simulink model "sistema_completo"  (R2019a)
settings: Solver=VariableStepAuto  StartTime=0.0  StopTime=120  RelTol=1e-3
InitFcn:
  | parametros
values from neighbouring files (symbols this model uses):
  a_h_max = 0.75    [parametros.m]
  a_t_max = 0.8    [parametros.m]
  b_cx = 1.0e6    (= 1000000)    [parametros.m]
  b_cy = 1.0e7    (= 10000000)    [parametros.m]
  b_h_eq = 2 * ( b_hd + i_h^2*b_hm ) / (r_hd^2)    (= 31004.4444444)    [parametros.m]
  b_hb = 1.0e8    (= 100000000)    [parametros.m]
  b_hEb = 2.2e9    (= 2200000000)    [parametros.m]
  b_t = 90.0    (= 90)    [parametros.m]
  b_t_eq = Simulink.Parameter(b_t_eq)    [parametros.m]
  b_tb = 5.0e6    (= 5000000)    [parametros.m]
  b_td_eq = ( b_td + i_t^2*b_tm ) / (r_td^2)    (= 21607.2)    [parametros.m]
  b_tw = 3.0e3    (= 3000)    [parametros.m]
  b_wu = 150    [parametros.m]
  clearance_min = 2    [parametros.m]
  g = Simulink.Parameter(9.80665)    [parametros.m]
  H_c = Simulink.Parameter(2.59)    [parametros.m]
  i_h = 22.0    (= 22)    [parametros.m]
  i_t = 30.0    (= 30)    [parametros.m]
  K_cy = 1.8e9    (= 1800000000)    [parametros.m]
  K_d_h = 2*m_h_eq*xi_hc*w_hc + m_h_eq*p3_hc - b_h_eq    (= 221460.31746)    [parametros.m]
  K_d_t = 2*m_t_eq*xi_tc*w_tc + m_t_eq*p3_tc - b_t_eq.Value    [parametros.m]
  K_i_h = m_h_eq*p3_hc*w_hc^2    (= 25598.9338431)    [parametros.m]
  K_i_t = m_t_eq*p3_tc*w_tc^2    [parametros.m]
  k_p3_th = 3    [parametros.m]
  K_p_h = m_h_eq*w_hc^2 + 2*m_h_eq*xi_hc*w_hc*p3_hc    (= 112940.617295)    [parametros.m]
  K_p_t = m_t_eq*w_tc^2 + 2*m_t_eq*xi_tc*w_tc*p3_tc    [parametros.m]
  k_th = 1    [parametros.m]
  K_tw = 4.8e5    (= 480000)    [parametros.m]
  k_w_c_th = 0.7    [parametros.m]
  k_wu = 2.36e8    (= 236000000)    [parametros.m]
  l_h0 = Y_t0 - y_h0    [parametros.m]
  L_h0 = 110    [parametros.m]
  l_h_man_thresh = 1.0    (= 1)    [parametros.m]
  l_h_tol = 1.0    (= 1)    [parametros.m]
  M_c_max = 50000    [parametros.m]
  M_c_min = 2000    [parametros.m]
  m_h_eq = 2 * ( J_hd_hEb + i_h^2*J_hm_hb ) / (r_hd^2)    (= 65137.7777778)    [parametros.m]
  M_s = 15000    [parametros.m]
  M_t = Simulink.Parameter(30000)    [parametros.m]
  m_td_eq = ( J_td + i_t^2*J_tm_tb ) / (r_td^2)    (= 30000)    [parametros.m]
  N_slots = Simulink.Parameter(floor((x_t_max_oper.Value - x_t_min_oper.Value) / W_c.Value))    [parametros.m]
  overload = false    [parametros.m]
  P_h_nom = 956150    [parametros.m]
  r_hd = 0.75    [parametros.m]
  r_td = 0.50    (= 0.5)    [parametros.m]
  random_obstacles = false    [parametros.m]
  T_hb_max = 5.0e4    (= 50000)    [parametros.m]
  T_hEb_max = 1.1e6    (= 1100000)    [parametros.m]
  T_hm_MAX = 2.0e4    (= 20000)    [parametros.m]
  T_s1 = 20/1000    (= 0.02)    [parametros.m]
  T_s2 = 1/1000    (= 0.001)    [parametros.m]
  T_tb_max = 5.0e3    (= 5000)    [parametros.m]
  T_tm_max = 4.0e3    (= 4000)    [parametros.m]
  tau_hm = 1.0    (= 1)    [parametros.m]
  tau_tm = 1.0    (= 1)    [parametros.m]
  v_h_max = 3.0    (= 3)    [parametros.m]
  v_h_nom = 1.5    [parametros.m]
  v_t_max = 4.0    (= 4)    [parametros.m]
  W_c = Simulink.Parameter(2.44)    [parametros.m]
  w_hm_rated = 2 * (i_h / r_hd) * v_h_nom    (= 88)    [parametros.m]
  x_l0 = x_t0    [parametros.m]
  x_t0 = W_c.Value / 2    [parametros.m]
  x_t_man_thresh = 1.0    (= 1)    [parametros.m]
  x_t_max_emer = x_t_max_oper.Value + 1.0    [parametros.m]
  x_t_max_oper = Simulink.Parameter(50.0)    [parametros.m]
  x_t_min_emer = x_t_min_oper.Value - 1.0    [parametros.m]
  x_t_min_oper = Simulink.Parameter(-30.0)    [parametros.m]
  x_td0 = x_t0    [parametros.m]
  xi_c_th = 0.7    [parametros.m]
  y_c0_0 = Simulink.Parameter(y_c0_ship)    [parametros.m]
  y_c0_quay = 0    [parametros.m]
  y_c0_ship = -20    [parametros.m]
  y_h_max_emer = y_h_max_oper.Value + 1.0    [parametros.m]
  y_h_max_oper = Simulink.Parameter(40.0)    [parametros.m]
  y_h_min_emer = y_h_min_oper.Value - 1.0    [parametros.m]
  y_h_min_oper = Simulink.Parameter(-20.0)    [parametros.m]
  y_l0 = y_h0    [parametros.m]
  Y_t0 = 45.0    (= 45)    [parametros.m]
undefined symbols (not defined in the file or in its folder): DiscIntNeverNeededParam, F_hw, hoist, l_h, l_h_dot, sigbuilder_block, theta_l, theta_l_dot, TLK, translation, x_t_dot
libraries: simulink x10, vrlib x1
(part 2 of 2)

== system sistema_completo/Planta física/Izaje del carro/Variables de estado derivadas ==
  note: Velocidad angular del tambor
  note: Caja reductora
      | entre motor y tambor
  note: Velocidad angular del motor
  note: Velocidad de despliegue del cable de izaje
  note: Longitud de cable de izaje desplegado
  note: Posición angular del motor
  note: Caja reductora
      | entre motor y tambor
  note: Radio del tambor
  note: Radio del tambor
  note: Normalizar ángulo en
      | rango 0 a 2*pi
  note: Posición angular del tambor
  note: Altura de carro (fija)
  note: Altura de la carga sin balanceo
  l_h_dot : Inport
  l_h : Inport  Port=2
  Constant1 : Constant  Value=2*pi
  Constant2 : Constant  Value=Y_t0
  Gain1 : Gain  Gain=-2/r_hd
  Gain2 : Gain  Gain=-2/r_hd
  Gain3 : Gain  Gain=i_h
  Gain4 : Gain  Gain=i_h
  Mod2 : Math  Operator=mod  SaturateOnIntegerOverflow=on
  Sum : Sum  Inputs=+-|
  w_hm : Outport
  w_hd : Outport  Port=2
  theta_hm : Outport  Port=3
  theta_hd : Outport  Port=4
  y_h : Outport  Port=5
  wires:
  Gain1/1 -> w_hd/1, Gain3/1  "w_hd"
  l_h_dot/1 -> Gain1/1
  Gain3/1 -> w_hm/1  "w_hm"
  Gain2/1 -> theta_hd/1, Gain4/1  "theta_hd"
  l_h/1 -> Sum/2, Gain2/1
  Gain4/1 -> Mod2/1  "theta_hm_raw"
  Constant1/1 -> Mod2/2
  Mod2/1 -> theta_hm/1
  Constant2/1 -> Sum/1
  Sum/1 -> y_h/1  "y_h"

== system sistema_completo/Planta física/Traslación del carro/Fines de carrera (fijos en viga) ==
  note: Posición horizontal del carro
  note: Fin de carrera de operación de límite normal mínimo
  note: Fin de carrera de operación de límite normal máximo
  note: Fin de carrera de emergencia de límite último mínimo
  note: Fin de carrera de operación de límite último máximo
  x_t : Inport
  Compare To Constant : simulink/Logic and Bit Operations/Compare To Constant  relop=<=  const=x_t_min_oper  OutDataTypeStr=boolean
  Compare To Constant1 : simulink/Logic and Bit Operations/Compare To Constant  relop=>=  const=x_t_max_oper  OutDataTypeStr=boolean
  Compare To Constant2 : simulink/Logic and Bit Operations/Compare To Constant  relop=<=  const=x_t_min_emer  OutDataTypeStr=boolean
  Compare To Constant3 : simulink/Logic and Bit Operations/Compare To Constant  relop=>=  const=x_t_max_emer  OutDataTypeStr=boolean
  x_t_min_oper : Outport  OutDataTypeStr=boolean  PortDimensions=1  SampleTime=0
  x_t_max_oper : Outport  Port=2  OutDataTypeStr=boolean  PortDimensions=1  SampleTime=0
  x_t_min_emer : Outport  Port=3  OutDataTypeStr=boolean  PortDimensions=1  SampleTime=0
  x_t_max_emer : Outport  Port=4  OutDataTypeStr=boolean  PortDimensions=1  SampleTime=0
  wires:
  Compare To Constant2/1 -> x_t_min_emer/1
  Compare To Constant/1 -> x_t_min_oper/1
  Compare To Constant1/1 -> x_t_max_oper/1
  x_t/1 -> Compare To Constant3/1, Compare To Constant2/1, Compare To Constant1/1, Compare To Constant/1
  Compare To Constant3/1 -> x_t_max_emer/1

== system sistema_completo/Planta física/Traslación del carro/Fuerza del cable del carro ==
  note: Posición de tambor del carro
  note: Velocidad del tambor del carro
  note: Posición del carro
  note: Velocidad del carro
  note: Fuerza del cable del carro
  x_td : Inport
  x_t : Inport  Port=2
  x_td_dot : Inport  Port=3
  x_t_dot : Inport  Port=4
  Gain : Gain  Gain=K_tw
  Gain1 : Gain  Gain=b_tw
  Sum2 : Sum  Inputs=+-
  Sum3 : Sum  Inputs=+-
  Sum4 : Sum
  F_tw : Outport
  wires:
  x_td_dot/1 -> Sum3/1
  x_td/1 -> Sum2/1
  x_t_dot/1 -> Sum3/2
  x_t/1 -> Sum2/2
  Sum4/1 -> F_tw/1
  Gain/1 -> Sum4/1
  Sum2/1 -> Gain/1
  Gain1/1 -> Sum4/2
  Sum3/1 -> Gain1/1

== system sistema_completo/Planta física/Traslación del carro/Fuerza motriz de tambor de carro equivalente ==
  note: Fuerza motriz de tambor
      | de carro equivalente
  note: Torque motor carro
  note: Freno eje rápido izaje
      | (operación)
  note: Estado de freno de
      | operación de carro
      | (eje rápido)
  note: Velocidad angular
      | del motor de carro
      | (eje rápido)
  T_tm : Inport
  BRK_t : Inport  Port=2  OutDataTypeStr=boolean
  w_tm : Inport  Port=3
  Constant4 : Constant  Value=-T_tb_max
  Constant5 : Constant  Value=T_tb_max
  Constant6 : Constant  Value=0
  Gain4 : Gain  Gain=i_t/r_td
  Gain7 : Gain  Gain=-b_tb
  MinMax2 : MinMax  Inputs=2
  MinMax3 : MinMax  Function=max  Inputs=2
  Sum1 : Sum  Inputs=++|
  Switch1 : Switch  Criteria=u2 ~= 0
  F_td_m_eq : Outport
  wires:
  MinMax3/1 -> MinMax2/2
  MinMax2/1 -> Switch1/3  "BRK_t = Off"
  Constant4/1 -> MinMax3/1
  T_tm/1 -> Sum1/1
  w_tm/1 -> Gain7/1
  Constant5/1 -> MinMax2/1
  Gain7/1 -> MinMax3/2
  BRK_t/1 -> Switch1/2
  Constant6/1 -> Switch1/1  "BRK_t = On"
  Sum1/1 -> Gain4/1
  Switch1/1 -> Sum1/2  "T_tb"
  Gain4/1 -> F_td_m_eq/1

== system sistema_completo/Planta física/Traslación del carro/Modulador de torque en accionamiento de carro ==
  note: Modelo de torque idealizado equivalente,
      | modelo simplificado de primer orden LTI en tiempo continuo
  note: Consigna de torque de motor de carro
  note: Torque de motor de carro
  T_tm* : Inport
  Gain1 : Gain  Gain=1/tau_tm
  Gain3 : Gain  Gain=-1
  Integrator2 : Integrator
  Limitador de torque máximo en tiempo discretizado : Subsystem
  Sum : Sum  Inputs=|++
  T_tm : Outport
  wires:
  Sum/1 -> Gain1/1
  Gain3/1 -> Sum/2
  Gain1/1 -> Integrator2/1  "T_tm_dot"
  Limitador de torque máximo en tiempo discretizado/1(T_tm_lim*) -> Sum/1  "T_tm_lim*"
  T_tm*/1 -> Limitador de torque máximo en tiempo discretizado/1(T_tm*)
  Integrator2/1 -> T_tm/1, Gain3/1  "T_tm"

== system sistema_completo/Planta física/Traslación del carro/Variables de estado derivadas ==
  note: Normalizar ángulo en
      | rango 0 a 2*pi
  note: Radio del tambor
  note: Caja reductora
      | entre motor y tambor
  note: Velocidad angular del motor del carro
  note: Velocidad de la carga sin balanceo
  note: Posición angular del motor del carro
  note: Caja reductora
      | entre motor y tambor
  note: Radio del tambor
  note: Posición horizontal
      | del tambor del carro
  x_td_dot : Inport
  x_td : Inport  Port=2
  Constant : Constant  Value=2*pi
  Gain1 : Gain  Gain=1/r_td
  Gain2 : Gain  Gain=1/r_td
  Gain3 : Gain  Gain=i_t
  Gain4 : Gain  Gain=i_t
  Mod1 : Math  Operator=mod  SaturateOnIntegerOverflow=on
  w_tm : Outport
  theta_tm : Outport  Port=2
  wires:
  Gain1/1 -> Gain3/1  "w_td"
  x_td_dot/1 -> Gain1/1
  Gain3/1 -> w_tm/1  "w_tm"
  x_td/1 -> Gain2/1
  Gain2/1 -> Gain4/1  "theta_td"
  Gain4/1 -> Mod1/1  "theta_tm_raw"
  Mod1/1 -> theta_tm/1
  Constant/1 -> Mod1/2

== system sistema_completo/Controladores de movimiento/Controladores de movimiento (Nivel 2)/Controlador de ángulo de balanceo/Des-linearización por retroalimentación ==
  note: Linearización por retroalimentación (feedback linearization)
      | F_t_eq = ( v - a ) / b
      | Siendo v la entrada virtual al sistema lineal a controlar
  m_l : Inport
  v : Inport  Port=2
  theta : Inport  Port=3
  theta_dot : Inport  Port=4
  x_t_dot : Inport  Port=5
  l_h : Inport  Port=6
  Add : Sum  Inputs=+-
  Divide : Product  Inputs=*/
  MATLAB Function : MATLAB Function  TreatAsAtomicUnit=on
  MATLAB Function1 : MATLAB Function  TreatAsAtomicUnit=on
  F_t_eq : Outport
  wires:
  Add/1 -> Divide/1
  v/1 -> Add/1
  Divide/1 -> F_t_eq/1
  MATLAB Function/1(a) -> Add/2
  MATLAB Function1/1(b) -> Divide/2
  theta/1 -> MATLAB Function1/1(theta), MATLAB Function/1(theta)
  theta_dot/1 -> MATLAB Function/2(theta_dot)
  x_t_dot/1 -> MATLAB Function/3(x_t_dot)
  l_h/1 -> MATLAB Function1/2(l_h), MATLAB Function/4(l_h)
  m_l/1 -> MATLAB Function/5(m_l), MATLAB Function1/3(m_l)

== system sistema_completo/Controladores de movimiento/Controladores de movimiento (Nivel 2)/Controlador de ángulo de balanceo/Ganancias programadas ==
  note: Ganancia proporcional K_p_th
      | K_p_th = w_c_th^2 + 2*xi_c_th*w_c_th*p3_th
  note: Ganancia derivativa K_d_th
      | K_d_th = 2*xi_c_th*w_c_th + p3_th
  note: Ganancia integral K_i_th
      | K_i_th = p3_th*w_c_th^2
  l_h : Inport
  Add : Sum
  Add1 : Sum
  Gain : Gain  Gain=2*xi_c_th
  Gain1 : Gain  Gain=2*xi_c_th
  Parametros deseados sistema a lazo cerrado : Subsystem
  Product : Product
  Product1 : Product
  Product2 : Product  Inputs=3
  K_p_th : Outport
  K_i_th : Outport  Port=2
  K_d_th : Outport  Port=3
  wires:
  l_h/1 -> Parametros deseados sistema a lazo cerrado/1(l_h)
  Parametros deseados sistema a lazo cerrado/1(w_c_th) -> Product2/3, Product2/2, Product/2, Product/1, Product1/1, Gain1/1
  Parametros deseados sistema a lazo cerrado/2(p3_th) -> Product2/1, Product1/2, Add1/2
  Product1/1 -> Gain/1
  Gain/1 -> Add/2
  Product/1 -> Add/1
  Add/1 -> K_p_th/1  "K_p_th"
  Gain1/1 -> Add1/1
  Add1/1 -> K_d_th/1  "K_d_th"
  Product2/1 -> K_i_th/1  "K_i_th"

== system sistema_completo/Planta física/Carga suspendida/Parámetros de carga/Generate random load  ==
  note: Masa de contenedor
      | Condiciones nominales: M_c_min <= M_cx <= M_c_max
      | Condición de sobrecarga: M_cx > M_c_max
  note: Condición de sobrecarga
  note: Masa del contenedor y carga
  note: Se actualiza la masa del contenedor de carga
      | cuando se cierran los twistlocks (TL K ↑)
  Trigger : TriggerPort  VariantControl=Variant  PortDimensions=1
  Constant : Constant  Value=M_c_min
  Constant1 : Constant  Value=M_c_max
  Constant2 : Constant  Value=1.25 * M_c_max
  Constant4 : Constant  Value=M_c_max
  MATLAB Function : MATLAB Function  TreatAsAtomicUnit=on
  Switch1 : Switch  Criteria=u2 ~= 0
  Switch2 : Switch  Criteria=u2 ~= 0
  h_c5 : Constant  Value=overload
  M_cx : Outport  OutDataTypeStr=double  PortDimensions=1  InitialOutput=0
  wires:
  MATLAB Function/1(y) -> M_cx/1
  Constant/1 -> Switch1/3
  Constant1/1 -> Switch1/1
  Constant2/1 -> Switch2/1
  Constant4/1 -> Switch2/3
  h_c5/1 -> Switch1/2, Switch2/2
  Switch1/1 -> MATLAB Function/1(min)
  Switch2/1 -> MATLAB Function/2(max)

== system sistema_completo/Planta física/Izaje del carro/Modulador de torque en accionamiento de izaje/Limitador de torque máximo en tiempo discretizado ==
  note: Torque de motor de izaje máximo
      | con reducción cuadrática
  note: Consigna de torque de motor de izaje
  note: Consigna de torque de motor de izaje
      | con limitación de torque máximo
  note: Modelo discretizado
      | k * T_s2 <= t < (k+1) * T_s2
  T_hm_max : Inport
  T_hm* : Inport  Port=2
  Gain : Gain  Gain=-1
  MinMax : MinMax  Inputs=2
  MinMax1 : MinMax  Function=max  Inputs=2
  Zero-Order Hold : ZeroOrderHold  SampleTime=T_s2
  Zero-Order Hold1 : ZeroOrderHold  SampleTime=T_s2
  T_hm_lim* : Outport
  wires:
  T_hm*/1 -> Zero-Order Hold/1
  MinMax/1 -> Zero-Order Hold1/1
  T_hm_max/1 -> MinMax/1, Gain/1
  Gain/1 -> MinMax1/1
  MinMax1/1 -> MinMax/2
  Zero-Order Hold/1 -> MinMax1/2
  Zero-Order Hold1/1 -> T_hm_lim*/1

== system sistema_completo/Planta física/Izaje del carro/Modulador de torque en accionamiento de izaje/Reducción cuadrática de torque máximo (field weakening) ==
  note: Velocidad del motor de izaje
  note: Velocidad del motor de izaje equivalente
      | para velocidad de izaje nominal
  note: Torque de motor de izaje máximo
      | con reducción cuadrática
  note: Torque de motor de izaje máximo
      | para velocidades menores o igual
      | a la velocidad nominal del motor
  w_hm : Inport
  Constant1 : Constant  Value=w_hm_rated
  Constant2 : Constant
  Divide : Product  Inputs=*/  SaturateOnIntegerOverflow=on
  Gain : Gain  Gain=T_hm_MAX
  MinMax : MinMax  Inputs=2
  Square : Math  Operator=square  SaturateOnIntegerOverflow=on
  T_hm_max : Outport
  wires:
  Constant2/1 -> MinMax/1
  MinMax/1 -> Gain/1
  Gain/1 -> T_hm_max/1
  w_hm/1 -> Divide/2
  Constant1/1 -> Divide/1
  Divide/1 -> Square/1
  Square/1 -> MinMax/2

== system sistema_completo/Planta física/Traslación del carro/Modulador de torque en accionamiento de carro/Limitador de torque máximo en tiempo discretizado ==
  note: Consigna de torque de motor de carro
  note: Consigna de torque de motor de carro
      | con limitación de torque máximo
  note: Modelo discretizado
      | k * T_s2 <= t < (k+1) * T_s2
  T_tm* : Inport
  Constant1 : Constant  Value=-T_tm_max
  Constant2 : Constant  Value=T_tm_max
  MinMax : MinMax  Inputs=2
  MinMax1 : MinMax  Function=max  Inputs=2
  Zero-Order Hold : ZeroOrderHold  SampleTime=T_s2
  Zero-Order Hold1 : ZeroOrderHold  SampleTime=T_s2
  T_tm_lim* : Outport
  wires:
  T_tm*/1 -> Zero-Order Hold/1
  MinMax/1 -> Zero-Order Hold1/1
  Constant1/1 -> MinMax1/1
  MinMax1/1 -> MinMax/2
  Zero-Order Hold/1 -> MinMax1/2
  Zero-Order Hold1/1 -> T_tm_lim*/1
  Constant2/1 -> MinMax/1

== system sistema_completo/Controladores de movimiento/Controladores de movimiento (Nivel 2)/Controlador de ángulo de balanceo/Ganancias programadas/Parametros deseados sistema a lazo cerrado ==
  note: Largo del cable de izaje
  note: Tercer polo de sistema a lazo cerrado
  note: Frecuencia natural del sistema a lazo cerrado
  l_h : Inport
  Constant : Constant  Value=k_w_c_th*sqrt(g)
  Divide : Product  Inputs=*/
  Gain : Gain  Gain=k_p3_th
  Sqrt : Sqrt  SaturateOnIntegerOverflow=on
  w_c_th : Outport
  p3_th : Outport  Port=2
  wires:
  Constant/1 -> Divide/1
  l_h/1 -> Sqrt/1
  Divide/1 -> w_c_th/1, Gain/1
  Sqrt/1 -> Divide/2
  Gain/1 -> p3_th/1

== matlab function sistema_completo/Planta física/Carga suspendida/Perfil de obstáculos/MATLAB Function ==
  data: x_l input; y_c0_x_l output; TLK input; y_c0 output size=[1, 1651]; x_t_min_oper parameter double size=1; W_c parameter double size=1; H_c parameter double size=1; y_c0_quay parameter double size=1; y_c0_ship parameter; random_obstacles parameter; N_slots parameter
function [y_c0_x_l,y_c0] = update_perfil_obstactulos(x_l, TLK, x_t_min_oper, W_c, H_c, y_c0_quay, y_c0_ship, random_obstacles, N_slots)
    % Actualiza el perfil de obstaculos con resolución de un slot por contenedor.
    % Entradas:
    % 1) x_l: posición horizontal del spreader [m]
    % 2) TLK: estado twistlocks [bool]
    % 3) N_slots: número de slots que caben en el rango de operación [-]
    % 4) x_t_min_oper: límite izquierdo de operación [m]
    % 5) W_c: ancho de contenedor [m]
    % 6) H_c: altura de contenedor [m]
    % 7) y_c0_quay: altura base del perfil en muelle [m]
    % 8) y_c0_ship: altura base del perfil en barco [m]
    % 9) random_obstacles: si true, inicializa con contenedores aleatoreos
    % Salidas:
    % 1) y_c0_x_l: perfil de obstáculo para la posición y tiempo actual [m]
    % 2) y_c0: vector perfil de obstáculos para el tiempo actual [m]

    persistent y_c0_prev;
    
    % Posicion (borde izquierdo) de cada slot, para saber si cae en muelle o barco
    x_slots = x_t_min_oper + (0:N_slots-1) * W_c;

    if isempty(y_c0_prev)
        % Inicializar y_c0_prev si es la primera ejecución
        y_c0_prev = zeros(1, N_slots);
        y_c0_prev(x_slots <  0) = y_c0_quay; % altura base lado muelle (x < 0)
        y_c0_prev(x_slots >= 0) = y_c0_ship; % altura base lado barco  (x >= 0)
        
        if random_obstacles
            % Número aleatorio de contenedores apilados por slot (0 a 10)
            n_max_stack = 10;
            for i = 1:N_slots
                n_stack = randi([0, n_max_stack]);
                y_c0_prev(i) = y_c0_prev(i) + n_stack * H_c;
            end
        end
    end
    
    % Índice del slot correspondiente a x_l
    % Cualquier posición dentro del slot lo activa
    slot_x_l = floor((x_l - x_t_min_oper) / W_c) + 1;
    slot_x_l = max(1, min(N_slots, slot_x_l));  % asegura rango válido
    
    % Actualizar y_c0 para slot correspondiente a x_l
    y_c0 = y_c0_prev; % Empieza con valores previos

    if (TLK)  % Si se cierran los twistlocks (se agarra el contenedor)
        y_c0(slot_x_l) = y_c0(slot_x_l) - H_c;
    else      % Si se abren los twistlocks (se suelta el contenedor)
        y_c0(slot_x_l) = y_c0(slot_x_l) + H_c;
    end
    
    % Buscar índice para x más cercano a x_l
    y_c0_x_l = y_c0(slot_x_l); % Actualiza valor de y_c0(x_l)
    
    % Guardar los valores actuales como previos para próxima iteración
    y_c0_prev = y_c0;
end

== matlab function sistema_completo/Planta física/Carga suspendida/Parámetros de carga/Generate random load /MATLAB Function ==
  data: y output; min input; max input
function y = update_random(min, max)
    persistent r;
    if isempty(r)
        rng('shuffle'); % Shuffle the seed ONCE at the start
    end
    r = randi([min, max]); % Generate a new random integer on trigger
    y = r;
end

== matlab function sistema_completo/Controladores de movimiento/Controladores de movimiento (Nivel 2)/Controlador de ángulo de balanceo/Des-linearización por retroalimentación/MATLAB Function ==
  data: theta input; a output; theta_dot input; x_t_dot input; l_h input; m_l input; g parameter double size=1; b_t_eq parameter double size=1; M_t parameter double size=1
function a = fcn(theta, theta_dot, x_t_dot, l_h, m_l, g, b_t_eq, M_t)
cos_theta = cos(theta);
sin_theta = sin(theta);

aux1 = m_l*g*sin_theta*cos_theta + m_l*l_h*sin_theta*theta_dot^2 - b_t_eq*x_t_dot;
aux2 = l_h*( M_t + m_l*sin_theta^2 );

a = -cos_theta * aux1 / aux2 - g*sin_theta/l_h;

== matlab function sistema_completo/Controladores de movimiento/Controladores de movimiento (Nivel 2)/Controlador de ángulo de balanceo/Des-linearización por retroalimentación/MATLAB Function1 ==
  data: theta input; b output; l_h input; m_l input; M_t parameter double size=1
function b = fcn(theta, l_h, m_l, M_t)
cos_theta = cos(theta);
sin_theta = sin(theta);

b = -cos_theta / ( l_h*( M_t + m_l*sin_theta^2 ) );

== stateflow chart sistema_completo/Controladores de movimiento/Control supervisor global (Nivel 1) ==
  state OPERATION [parallel]
    during:
    settings: executionOrder=1
    state INIT
      entry:
      %% INICIALIZA VARIABLES
      % Frenos
      % false: freno desenergizado, cerrado, hay torque de fricción
      % true: freno energizado, abierto, no hay torque de fricción
      BRK_t = true;     % freno de operación del carro
      BRK_h = true;    % freno de operación de izaje
      %BRK_hE = true;  % freno de emergencia de izaje
      % Twistlocks
      % false: twistlocks abiertos, spreader vacío (sin container)
      % true: twistlocks cerrados, spreader cargado (con container)
      TLK_OUT = false;
      % Masa de carga estimada
      M_cx = 0; % masa del spreader
      % Velocidades de referencia
      v_t_ref=0;
      v_h_ref=0;
    state IDLE
      entry:
    state FAULT [commented out]
      x=0;
    state OPERATIVE
      during:
      state MANUAL
        during:
        state LIFTOFF
          entry:
          v_h_ref = 0;  % [m/s] Velocidad de izaje de referencia
          v_h_ref_prev = 0;  % [m/s] Velocidad de izaje de referencia del paso previo
          v_h_ref_step = 0.001;  % [m/s] Rampa de velocidad de izaje
          flag_m_estim = true;  % [-] Flag de estimacion de masa de carga
          %M_cx = M_s;  % [kg] Masa de carga estimada (inicialmente igual a masa de spreader)
          F_hw_min = M_s * g / 2;  % [N] Fuerza de cable de izaje minima para estimacion de carga
          F_hw_prev = 0;  % [N] Fuerza del cable de izaje medido en paso previo
          F_hw_stable_tol = 0.009 * F_hw_min;  % [N] Tolerancia a diferencia de fuerza de izaje (0.9% carga minima)
          F_hw_stable = false;  % [-] Flag de fuerza de izaje estable
          F_hw_stable_cnt = 0;  % [-] Contador de pasos de fuerza de izaje estable
          F_hw_stable_cnt_min = 200; % [-] Pasos con fuerza de izaje estable necesarios para estimacion de carga
          TLK_prev = false; % [-] Estado de entrada de twistlock del paso previo
          during:
          % Freno de izaje debe estar energizado (sin torque de freno)
          % y el comando de izaje fuera de la zona muerta
          if (BRK_h==true && abs(command.hoist) > 0.1)
          % Izaje manual suave
          % Rampa hasta 10% de velocidad nominal segun input
          if (abs(v_h_ref) < abs(command.hoist * v_h_nom * 0.1))
          v_h_ref = v_h_ref_prev + sign(command.hoist) * v_h_ref_step;
          else
          v_h_ref = command.hoist * v_h_nom * 0.1;
          end
          else
          % Rampa de bajada a cero cuando comando liberado
          % 50% más rápido que cuando se comanda
          if (abs(v_h_ref_prev) > v_h_ref_step)
          v_h_ref = v_h_ref_prev - sign(v_h_ref_prev) * 1.5 * v_h_ref_step;
          else
          v_h_ref = 0;
          end
          end
          % Estimación de masa de carga cuando se estabiliza lectura
          % de fuerza de tensión del cable
          if (flag_m_estim && sensor.F_hw > 0.9*F_hw_min)
          if (abs(sensor.F_hw - F_hw_prev) < F_hw_stable_tol)
          if (F_hw_stable_cnt >= F_hw_stable_cnt_min)
          M_cx = 2 * sensor.F_hw / g;
          flag_m_estim = false;
          else
          F_hw_stable_cnt = F_hw_stable_cnt + 1;
          end
          else
          F_hw_stable_cnt = 0;
          end
          end
          % Deteccion de cable flojo: spreader totalmente apoyado sobre container
          % Cambio de modo de twistlocks solo en este estado
          if (sensor.F_hw < F_hw_stable_tol)
          % Deteccion flanco ascendente de entrada de twistlock
          if (TLK_prev == false && command.TLK == true)
          TLK_OUT = ~TLK_OUT;
          flag_m_estim = true; % reset flag of load estimation when the twistlocks state changes
          end
          end
          % Detección de nivel de modo automático
          % Sólo si la masa de la carga ha sido estimada
          if (flag_m_estim == false)
          % Y la altura de izaje supera zona segura
          if (sensor.l_h < 60)  % TODO: calcular nivel de modo automatico
          %send(EVT_AUTO);
          end
          end
          % Actualizar variables de valores previos
          v_h_ref_prev = v_h_ref;
          F_hw_prev = sensor.F_hw;
          TLK_prev = command.TLK;
          note: (DESPEGUE)
        (default) -> LIFTOFF
      state AUTOMATIC [commented out]
        during:
        state INIT_AUTO [commented out]
          entry:
          %% 1. Calcular distancia de izaje a recorrer
          % Calcular largo de cable de destino (considerando balanceo nulo)
          l_h_dest = Y_t0 - y_h_dest;
          % Número de slots que caben en el rango de operación
          N_slots = floor((x_t_max_oper - x_t_min_oper) / W_c);
          % Determinar slots activos de perfil de obstáculos: solo entre posición x actual y destino
          slot_cur   = max(1, min(N_slots, floor(sensor.x_t / W_c) + 1));
          slot_dest = max(1, min(N_slots, floor(x_t_dest    / W_c) + 1));
          slot_min  = min(slot_cur,  slot_dest);
          slot_max = max(slot_cur, slot_dest);
          % Altura pico del perfil entre posición x actual y destino
          y_h_peak = max(y_c0(slot_min:slot_max)) + clearance_min;
          l_h_peak  = Y_t0 - y_h_peak;
          % Calcular distancia de izaje: subida + bajada sobre el perfil
          % (no distancia directa origen-destino)
          d_h_up   = abs(l_h_peak - sensor.l_h);   % subida: posicion actual -> pico
          d_h_down = abs(l_h_peak - l_h_dest);   % bajada: pico -> destino
          d_h_total = d_h_up + d_h_down;
          %% 2. Calcular distancia horizontal a recorrer
          d_t_total  = abs(x_t_dest - sensor.x_t);  % [m] distancia en eje x
          %% 3. Calcular velocidad máxima de izaje (a potencia constante en función de la carga)
          % P_h_nom = m_l * g * v_h => v_h = P_h_nom / ( m_l * g )
          % No debe superar la velocidad máxima de izaje a carga nominal v_h_max
          v_h_max_load = min(v_h_max, P_h_nom / ( M_cx * g ));
          %% 4. Calcular tiempos de izaje y traslación
          % CASO 1: PERFIL TRAPEZOIDAL CON RAMPA SIMÉTRICA
          % T = t_ramp_up + t_cruise + t_ramp_down
          % Aceleración constante a_max en rampas
          % t_ramp_up = t_ramp_down = t_ramp = v_max / a_max
          % d_ramp = 1/2 * a_max * t_ramp^2 = v_max^2 / (2 * a_max)
          % Velocidad constante v_max en resto del tiempo
          % d_cruise = d_total - 2 * d_ramp = d_total - v_max^2 / a_max
          % t_cruise = d_cruise / v_max = (d_total / v_max) - (v_max / a_max)
          % Entonces, el tiempo total es
          % T = 2 * t_ramp + t_cruise = (2 * v_max / a_max) + (d_total / v_max) - (v_max / a_max)
          % T = v_max / a_max + d_total / v_max
          % CASO 2: PERFIL TRIANGULAR (distancia demasiado corta para alcanzar v_max)
          % T = t_ramp_up + t_ramp_down = 2 * t_ramp
          % d_total = 2 * d_ramp = 2 * (1/2 * a_max * t_ramp^2) = a_max * t_ramp^2
          % Entonces
          % t_ramp = sqrt(d_total / a_max)
          % Luego, el tiempo total es
          % T = 2 * sqrt(d_total / a_max)
          %% 4.1. Calcular tiempo de izaje
          % Distancia recorrida en rampas de subida y bajada para alcanzar velocidad v_h_max_load
          % a aceleración constante a_h_max
          d_ramp_total_h = v_h_max_load^2 / a_h_max
          % Tiempo de subida: posición actual l_h -> posición pico l_h_peak
          if (d_h_up >= d_ramp_total_h)  % trapezoidal
          T_h_up = v_h_max_load / a_h_max + d_h_up / v_h_max_load;
          else  % triangular
          T_h_up = 2 * sqrt(d_h_up / a_h_max);
          end
          % Tiempo de bajada: posición pico l_h_peak -> posición destino l_h_dest
          if (d_h_down >= d_ramp_total_h)  % trapezoidal
          T_h_down = v_h_max_load / a_h_max + d_h_down / v_h_max_load;
          else  % triangular
          T_h_down = 2 * sqrt(d_h_down / a_h_max);
          end
          % Tiempo total de izaje
          T_h = T_h_up + T_h_down;
          %% 4.2. Calcular tiempo de traslación
          d_ramp_total_t = v_t_max^2 / a_t_max;
          if (d_t_total >= d_ramp_total_t)  % trapezoidal
          T_t = v_t_max / a_t_max + d_t_total / v_t_max;
          else  % triangular
          T_t = 2 * sqrt(d_t_total / a_t_max);
          end
          %% 4.3. Eje más lento marca el tiempo total (sincronizacion de ejes)
          T_slow = max(T_h, T_t);
          %% 5. Calcular velocidades máximas sincronizadas (ambos ejes terminan simultáneamente)
          % Factores de escala: el eje rápido reduce su velocidad
          k_sync_h = T_h / T_slow;  % = 1 si izaje es el eje lento
          k_sync_t  = T_t  / T_slow;  % = 1 si traslación es el eje lento
          % Velocidades máximas sincronizadas
          v_h_max_sync = v_h_max_load * k_sync_h;
          v_t_max_sync  = v_t_max           * k_sync_t;
          %% 6. Generación de trayectoria terminada
          send(EVT_TRAJ_OK);
        state TRAVEL [commented out]
          state HOIST_AUTO [parallel] [commented out]
            entry:
            % Determinar fase de izaje basado en posición
            if (sensor.l_h > l_h_peak)
            % l_h > l_h_peak: necesitamos subir y luego bajar
            hoist_phase = 1;
            else
            % l_h <= l_h_peak: necesitamos bajar directamente
            hoist_phase = 2;
            end
            during:
            if (hoist_phase == 1)
            %% FASE 1: Subida hacia l_h_peak
            % (cable se acorta: v_h > 0)
            % Distancia remanente a l_h_peak
            dist_remaining_up = abs(sensor.l_h - l_h_peak);
            % Distancia de frenado desde velocidad actual a aceleración máxima
            d_brake_h = v_h_ref^2 / (2 * a_h_max);
            %% Comparar distancia necesaria para frenar con distancia remanente
            if (dist_remaining_up > d_brake_h)
            % Zona de aceleración o crucero
            v_h_ref = min(v_h_ref + a_h_max * T_s1, v_h_max_sync);
            else
            % Zona de desaceleración
            v_h_ref = max(v_h_ref - a_h_max * T_s1, 0);
            end
            % Transición a fase 2
            if (dist_remaining_up < l_h_tol || v_h_ref == 0)
            hoist_phase = 2;
            v_h_ref = 0;
            end
            else
            %% FASE 2: Bajada de l_h_peak a posición de destino l_h_dest
            % (cable se alarga: v_h < 0)
            % Distancia remanente a posición de destino
            dist_remaining_down = abs(sensor.l_h - l_h_dest);
            % Distancia de frenado desde velocidad actual a aceleración máxima
            d_brake_h = v_h_ref^2 / (2 * a_h_max);
            %% Comparar distancia necesaria para frenar con distancia remanente
            if (dist_remaining_down > d_brake_h + l_h_man_thresh)
            % Zona de aceleración o crucero (velocidad negativa = bajar)
            v_h_ref = max(v_h_ref - a_h_max * T_s1, -v_h_max_sync);
            else
            % Zona de desaceleración hacia zona manual
            v_h_ref = min(v_h_ref + a_h_max * T_s1, 0);
            end
            % Llegada a zona manual: pasar el control al operador
            if (dist_remaining_down < l_h_man_thresh)
            send(EVT_MANUAL);
            end
            end
            % Anomalía: cable flojo durante subida
            if (v_h_ref > 0 && sensor.F_hw < F_hw_slack_thr)
            send(EVT_SLACK_ROPE);
            end
            exit:
            v_h_ref_prev = v_h_ref;
          state TRANS_AUTO [parallel] [commented out]
            entry:
            dir_t = sign(x_t_dest - sensor.x_t);  % dirección hacia destino
            during:
            % Distancia remanente a posición de destino
            dist_remaining_t = abs(x_t_dest - sensor.x_t);
            % Distancia de frenado desde velocidad actual a aceleración máxima
            d_brake_t = v_t_ref^2 / (2 * a_t_max);
            % Comparar distancia necesaria para frenar con distancia remanente
            if (dist_remaining_t > d_brake_t + x_t_man_thresh)
            % Zona de aceleración o crucero
            v_t_ref = dir_t * min(abs(v_t_ref) + a_t_max * T_s1, v_t_max_sync);
            else
            % Zona de desaceleración hacia zona manual
            v_t_ref = dir_t * max(abs(v_t_ref) - a_t_max * T_s1, 0);
            end
            % Llegada a zona manual
            if (dist_remaining_t < x_t_man_thresh)
            send(EVT_MANUAL);
            end
            exit:
            v_t_ref_prev = v_t_ref;
        (default) -> INIT_AUTO [commented out]
        INIT_AUTO -> TRAVEL [commented out]
      (default) -> MANUAL
      AUTOMATIC -> MANUAL [commented out] : EVT_MANUAL
      MANUAL -> AUTOMATIC [commented out] : EVT_AUTO
    (default) -> INIT
    INIT -> IDLE
    FAULT -> IDLE [commented out]
    IDLE -> FAULT [commented out]
    IDLE -> OPERATIVE
    OPERATIVE -> FAULT [commented out]
  state MONITOR [parallel] [commented out]
    entry:
    zero_thres = 1; % [N] límite para detección de cable flojo
    disp('Entered MONITOR')
    during:
    % Cable de izaje flojo (carga apoyada)
    if sensor.F_hw < zero_thres
    %send(EVT_SLACK_ROPE);
    end
    % Sobrecarga
    if M_cx > M_c_max
    %send(EVT_OVERLOAD);
    end
    settings: description=|
        | Monitorea el estado de sistema:
        | - Detección de cable de izaje flojo
        | - Detección de sobrecarga
    note: % Sobrevelocidad de izaje: 15% sobre v_h_max
        |     %if abs(sensor.l_h_dot) > 1.15 * v_h_max
        |     %    send(EVT_OVERSPEED_H);
        |     %end
        |     % Sobrevelocidad de carro: 15% sobre v_t_max
        |     %if abs(sensor.x_t_dot) > 1.15 * v_t_max
        |     %    send(EVT_OVERSPEED_T);
        |     %end
  data: SensorBus local size=7; v_t_ref output; v_h_ref output; sensor input sensor_bus; command input command_bus; M_cx output double; TLK_OUT output; BRK_t output; BRK_h output; M_c_max parameter; v_h_max parameter; M_s parameter; v_h_nom parameter; g parameter; F_hw_stable local; F_hw_prev local; flag_m_estim local; v_h_ref_prev local; v_h_ref_step local; F_hw_stable_tol local; F_hw_stable_cnt local; zero_thres local; F_hw_stable_cnt_min local; F_hw_min local; TLK_prev local boolean; x_t_dest input; y_h_dest input; y_c0 input; W_c parameter; clearance_min parameter; P_h_nom parameter; v_t_max parameter; a_h_max parameter; a_t_max parameter; T_s1 parameter; hoist_phase local; x_t_man_thresh parameter; l_h_tol parameter; l_h_man_thresh parameter; v_h_max_sync local; v_t_max_sync local
  events: EVT_SLACK_ROPE local FUNCTION_CALL_EVENT; EVT_OVERSPEED_H local FUNCTION_CALL_EVENT; EVT_OVERSPEED_T local FUNCTION_CALL_EVENT; EVT_OVERLOAD local FUNCTION_CALL_EVENT; EVT_MANUAL local FUNCTION_CALL_EVENT; EVT_AUTO local FUNCTION_CALL_EVENT
